simulink model "zawieszenie_18"  (R2018a)
settings: Solver=ode4  StartTime=0.0  StopTime=20  FixedStep=0.01  RelTol=1e-3
values from neighbouring files (symbols this model uses):
  Alfa = X0(2)    [ident.m]    (also in zawieszenie_d.m = 123.1)
  Beta = X0(3)    [ident.m]    (also in zawieszenie_d.m = 0.125)
  cc = 15000    [zawieszenie_d.m]
  cw = 200000    [zawieszenie_d.m]
  dc = 200    [zawieszenie_d.m]
  dw = 10    [zawieszenie_d.m]
  k = X0(1)    [ident.m]    (also in zawieszenie_d.m = 1054)
  mc = 250    [zawieszenie_d.m]
  mw = 30    [zawieszenie_d.m]
  w0 = 0    [zawieszenie_d.m]
settings Model: Creator=Mariusz  LastModifiedBy=Mariusz
settings DataIOCC: ReturnWorkspaceOutputs=on
settings SFSimCC: SimUseLocalCustomCode=on
settings RTWCC: RTWUseLocalCustomCode=on

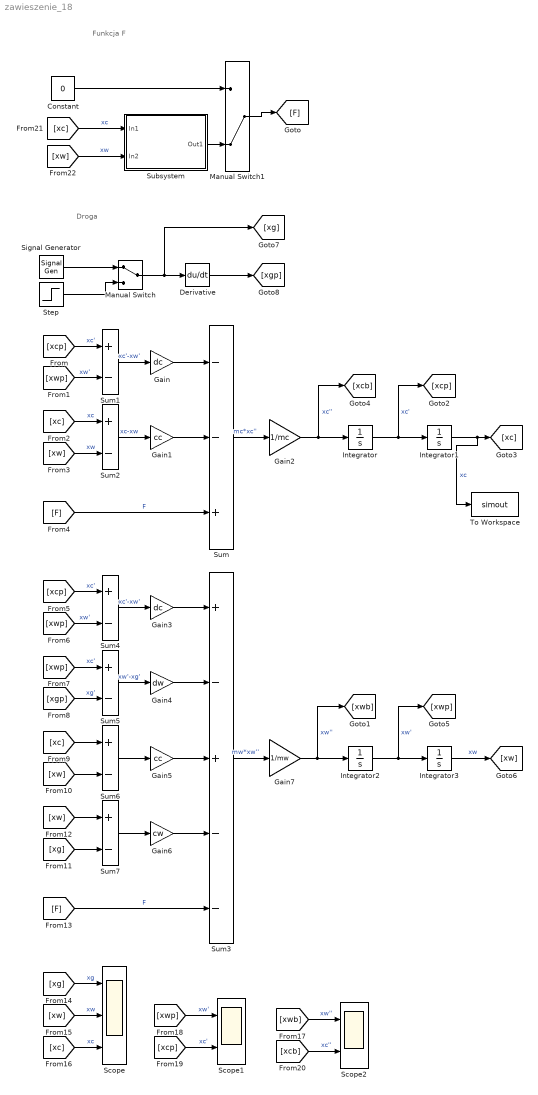
== system zawieszenie_18 ==
  note: Droga
  note: Funkcja F
  Constant : Constant  Value=0
  Derivative : Derivative
  Gain : Gain  Gain=dc
  Gain1 : Gain  Gain=cc
  Gain2 : Gain  Gain=1/mc
  Gain3 : Gain  Gain=dc
  Gain4 : Gain  Gain=dw
  Gain5 : Gain  Gain=cc
  Gain6 : Gain  Gain=cw
  Gain7 : Gain  Gain=1/mw
  Integrator{,1..3} (4 alike) : Integrator
  Manual Switch : ManualSwitch
  Manual Switch1 : ManualSwitch  CurrentSetting=0
  Scope : Scope  NumInputPorts=3
  Scope1 : Scope  NumInputPorts=2
  Scope2 : Scope  NumInputPorts=2
  Signal Generator : SignalGenerator  WaveForm=square  Amplitude=0.05  Frequency=0.5  Units=rad/sec
  Step : Step  Time=0  After=0.1  SampleTime=0
  Subsystem : Subsystem
  Sum : Sum  Inputs=--+
  Sum{1..2,4..7} (6 alike) : Sum  Inputs=+-
  Sum3 : Sum  Inputs=+-+--
  To Workspace : ToWorkspace  VariableName=simout  SaveFormat=Timeseries  SampleTime=-1
  wires:
  [xcp] -> Sum1/1  "xc'"
  [xwp] -> Sum1/2  "xw'"
  Sum1/1 -> Gain/1  "xc'-xw'"
  Gain/1 -> Sum/1
  Sum2/1 -> Gain1/1  "xc-xw"
  [xw] -> Sum2/2  "xw"
  [xc] -> Sum2/1  "xc"
  Gain1/1 -> Sum/2
  [F] -> Sum/3  "F"
  Constant/1 -> Manual Switch1/1
  Sum/1 -> Gain2/1  "mc*xc''"
  Integrator/1 -> [xcp], Integrator1/1  "xc'"
  Integrator1/1 -> To Workspace/1, [xc]  "xc"
  Sum4/1 -> Gain3/1  "xc'-xw'"
  [xwp] -> Sum4/2  "xw'"
  Gain3/1 -> Sum3/1
  [xcp] -> Sum4/1  "xc'"
  Sum5/1 -> Gain4/1  "xw'-xg'"
  [xgp] -> Sum5/2  "xg'"
  Gain4/1 -> Sum3/2
  [xwp] -> Sum5/1  "xc'"
  Sum6/1 -> Gain5/1
  [xw] -> Sum6/2
  Gain5/1 -> Sum3/3
  [xc] -> Sum6/1
  [xw] -> Sum7/1
  [xg] -> Sum7/2
  Sum7/1 -> Gain6/1
  Gain6/1 -> Sum3/4
  [F] -> Sum3/5  "F"
  Sum3/1 -> Gain7/1  "mw*xw''"
  Integrator2/1 -> [xwp], Integrator3/1  "xw'"
  Integrator3/1 -> [xw]  "xw"
  Derivative/1 -> [xgp]
  [xg] -> Scope/1  "xg"
  [xw] -> Scope/2  "xw"
  [xc] -> Scope/3  "xc"
  [xwp] -> Scope1/1  "xw'"
  [xcp] -> Scope1/2  "xc'"
  [xwb] -> Scope2/1  "xw''"
  [xcb] -> Scope2/2  "xc''"
  Gain7/1 -> [xwb], Integrator2/1  "xw''"
  Gain2/1 -> [xcb], Integrator/1  "xc''"
  Manual Switch/1 -> [xg], Derivative/1
  Step/1 -> Manual Switch/2
  Manual Switch1/1 -> [F]
  Subsystem/1(Out1) -> Manual Switch1/2
  [xc] -> Subsystem/1(In1)  "xc"
  [xw] -> Subsystem/2(In2)  "xw"
  Signal Generator/1 -> Manual Switch/1

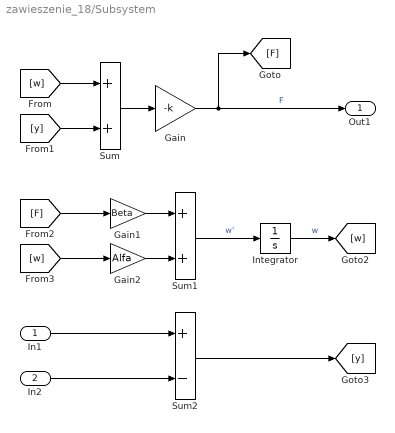
== system zawieszenie_18/Subsystem ==
  In1 : Inport
  In2 : Inport  Port=2
  Gain : Gain  Gain=-k
  Gain1 : Gain  Gain=Beta
  Gain2 : Gain  Gain=Alfa
  Integrator : Integrator  InitialCondition=w0
  Sum : Sum
  Sum1 : Sum
  Sum2 : Sum  Inputs=+-
  Out1 : Outport
  wires:
  [y] -> Sum/2
  Sum/1 -> Gain/1
  Gain/1 -> [F], Out1/1  "F"
  [F] -> Gain1/1
  [w] -> Gain2/1
  Gain1/1 -> Sum1/1
  Gain2/1 -> Sum1/2
  Sum1/1 -> Integrator/1  "w'"
  Integrator/1 -> [w]  "w"
  In1/1 -> Sum2/1
  In2/1 -> Sum2/2
  Sum2/1 -> [y]
  [w] -> Sum/1
